simulink model "L2f"  (R2022b)
settings: Solver=VariableStepAuto  StartTime=0.0  StopTime=10.0  RelTol=1e-3
settings Model: Creator=Milosh Yokich  LastModifiedBy=Milosh Yokich

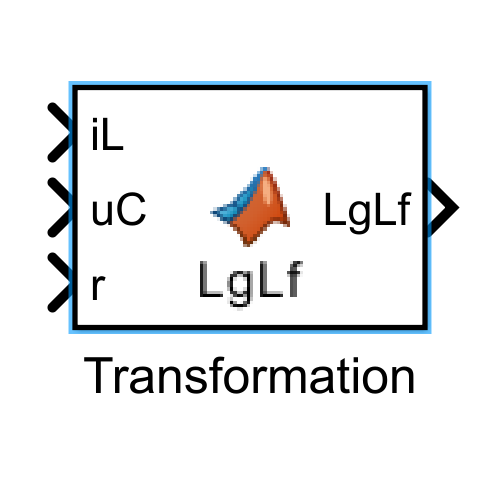
[thumbnail: Simulink's stored preview of the top-level diagram]
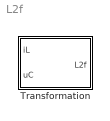
== system L2f ==
  Transformation : MATLAB Function  TreatAsAtomicUnit=on

== matlab function L2f/Transformation ==
  data: iL input; L2f output; uC input
function L2f = L2f(iL, uC)
E = 12; %V
R = 52; %Omh
L = 0.01591; %H
C = 0.000470; %F 

L2f = -E/L*uC + (1/C*iL + uC/(C*R))*(-E/R + 2*uC/R);
